simulink model "E_sim"  (R2017a)
settings: Solver=ode45  StartTime=0.0  StopTime=10000  MaxStep=.1  RelTol=1e-3  EnableMultiTasking=on
InitFcn:
  | addpath ./..
  | clear;clc
  | E_param
undefined symbols (not defined in the file or in its folder): E_animation
libraries: simulink x1
settings Model: Creator=beard  LastModifiedBy=Mat Haskell
settings DataIOCC: LimitDataPoints=on  SaveFormat=Array  SignalLoggingSaveFormat=ModelDataLogs
settings OptimizationCC: ExpressionDepthLimit=2147483647  InitFltsAndDblsToZero=on  LifeSpan=inf
settings DebuggingCC: UnderspecifiedInitializationDetection=Classic  MergeDetectMultiDrivingBlocksExec=none  SolverPrmCheckMsg=warning  FcnCallInpInsideContextMsg=warning  StateNameClashWarn=warning  SFUnexpectedBacktrackingDiag=warning  SFNoUnconditionalDefaultTransitionDiag=warning  SFExecutionAtInitializationDiag=none
settings HardwareCC: ProdBitPerPointer=32  ProdBitPerSizeT=32  ProdBitPerPtrDiffT=32  ProdLargestAtomicFloat=None  ProdIntDivRoundTo=Undefined  ProdEndianess=Unspecified  ProdWordSize=32  ProdHWDeviceType=32-bit Generic
settings ModelReferenceCC: PropagateSignalLabelsOutOfModel=off
settings GRTTargetCC: TargetLangStandard=C89/C90 (ANSI)  GeneratePreprocessorConditionals=Disable all  CombineOutputUpdateFcns=off  GRTInterface=on
settings ConfigComp: CovMetricSettings=dw  CovHtmlReporting=on  CovSaveCumulativeToWorkspaceVar=on  CovSaveSingleToWorkspaceVar=on  CovExternalEMLEnable=off

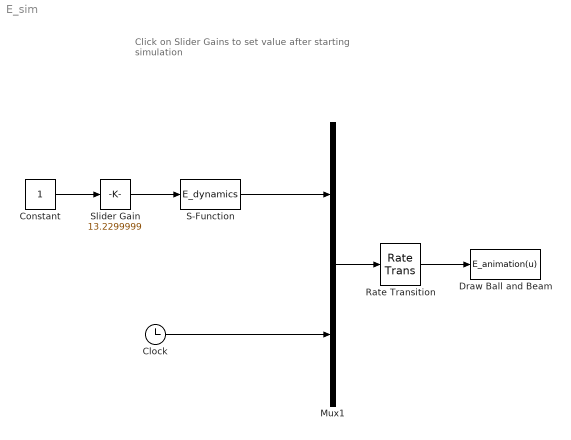
== system E_sim ==
  note: Click on Slider Gains to set value
      | after starting simulation
  Clock : Clock
  Constant : Constant
  Draw Ball and Beam : MATLABFcn  MATLABFcn=E_animation(u)  OutputDimensions=0
  Mux1 : Mux  Inputs=2
  Rate Transition : RateTransition  OutPortSampleTime=P.t_plot
  S-Function : S-Function  InitFcn=E_param  FunctionName=E_dynamics  Parameters=P  SFunctionDeploymentMode=off  EnableBusSupport=off
  Slider Gain : simulink/Math Operations/Slider Gain  gain=13.2299999  low=0  high=20
  wires:
  Clock/1 -> Mux1/2
  Mux1/1 -> Rate Transition/1
  Rate Transition/1 -> Draw Ball and Beam/1
  S-Function/1 -> Mux1/1
  Slider Gain/1 -> S-Function/1
  Constant/1 -> Slider Gain/1
